simulink model "y003"  (R2019b)
settings: Solver=ode23tb  StartTime=0.0  StopTime=1  MaxStep=0.00001  RelTol=1e-3
values from neighbouring files (symbols this model uses):
  band = 0.01    [parameter.m]
  fN = 50    [parameter.m]
  J = 0.1284    [parameter.m]
  Llr = Lr - Lm    (= 0.006)    [parameter.m]
  Lls = Ls - Lm    (= 0.0102)    [parameter.m]
  np = 2    [parameter.m]
  PN = 3000    [parameter.m]
  Rr = 2.685    [parameter.m]
  Rs = 1.85    [parameter.m]
  TN = PN/(2*pi*nN/60)    (= 20.4627783975)    [parameter.m]
  UN = 380    [parameter.m]
undefined symbols (not defined in the file or in its folder): i
libraries: powerlib x9, simulink x3
Description:
  | 直接使用转子磁链数据，电流滞环跟踪
settings Model: Creator=Inspiron  LastModifiedBy=Inspiron
settings SolverCC: ZeroCrossAlgorithm=Adaptive
settings DebuggingCC: IgnoredZcDiagnostic=none

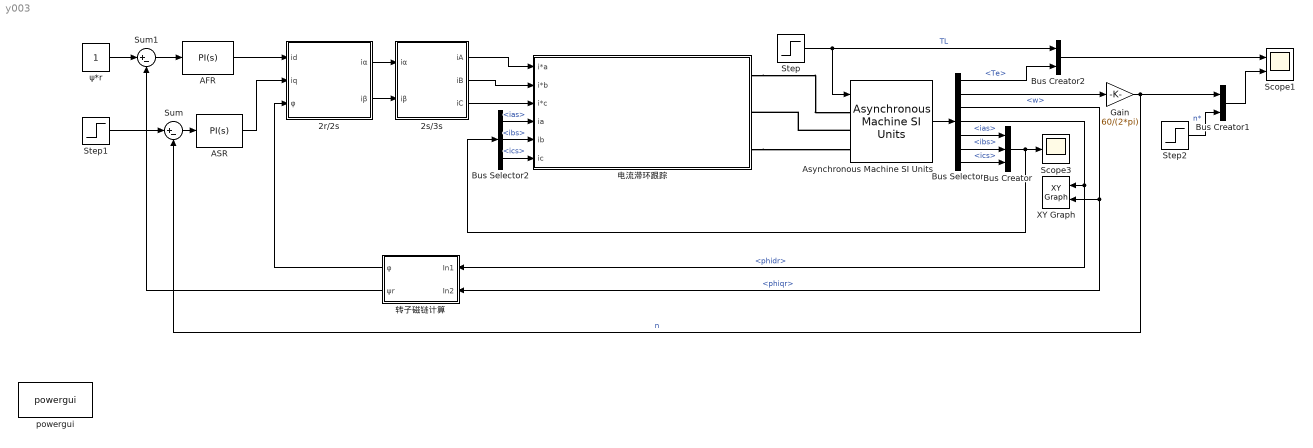
== system y003 ==
  2r/2s : Subsystem
  2s/3s : Subsystem
  AFR : simulink/Continuous/PID Controller  Controller=PI  Form=Parallel  TimeDomain=Continuous-time  SampleTime=-1  IntegratorMethod=Forward Euler  FilterMethod=Forward Euler  ControllerParametersSource=internal  P=80  I=20  D=0  UseFilter=on  N=100  TunerSelectOption=Transfer Function Based (PID Tuner App)  InitialConditionSource=internal  InitialConditionForIntegrator=0  InitialConditionForFilter=0  DifferentiatorICPrevScaledInput=0  ExternalReset=none  TrackingMode=off  Kt=1  LimitOutput=on  UpperSaturationLimit=40  LowerSaturationLimit=-40  LinearizeAsGain=on  AntiWindupMode=none  Kb=1  POutMin=[]  POutMax=[]  IOutMin=[]  IOutMax=[]  DOutMin=[]  DOutMax=[]  NOutMin=[]  NOutMax=[]  SumOutMin=[]  SumOutMax=[]  SaturationOutMin=[]  SaturationOutMax=[]  PParamMin=[]  PParamMax=[]  IParamMin=[]  IParamMax=[]  DParamMin=[]  DParamMax=[]  NParamMin=[]  NParamMax=[]  KbParamMin=[]  KbParamMax=[]  KtParamMin=[]  KtParamMax=[]  KbOutMin=[]  KbOutMax=[]  KtOutMin=[]  KtOutMax=[]  IntegratorOutMin=[]  IntegratorOutMax=[]  FilterOutMin=[]  FilterOutMax=[]  SumI1OutMin=[]  SumI1OutMax=[]  SumI2OutMin=[]  SumI2OutMax=[]  SumI3OutMin=[]  SumI3OutMax=[]  SumI4OutMin=[]  SumI4OutMax=[]  SumDOutMin=[]  SumDOutMax=[]  DifferentiatorOutMin=[]  DifferentiatorOutMax=[]  FilterDiffOutCoefMin=[]  FilterDiffOutCoefMax=[]  ReciprocalOutMin=[]  ReciprocalOutMax=[]  SumDenOutMin=[]  SumDenOutMax=[]  SumNumOutMin=[]  SumNumOutMax=[]  DivideOutMin=[]  DivideOutMax=[]  IntegratorContinuousStateAttributes=''  IntegratorStateMustResolveToSignalObject=off  IntegratorRTWStateStorageClass=Auto  FilterContinuousStateAttributes=''  FilterStateMustResolveToSignalObject=off  FilterRTWStateStorageClass=Auto  ParallelPVariant=InternalParameters  IdealPVariant=Disabled  IVariant=InternalParameters  DVariant=Disabled  IntegratorVariant=Continuous  SatVariant=Enabled  AWVariant=Passthrough  PCopyVariant=Disabled  TRVariant=Disabled  FdbkBlocksVariant=Forward  IdealPFdbkVariant=Disabled  SatFdbkVariant=Disabled  DerivativeFilterVariant=Disabled  NVariant=Disabled  NCopyVariant=Disabled_SignalSpec  FilterICVariant=Disabled  IntegratorICVariant=InternalICs  ExternalResetVariant=Disabled  TRSumVariant=Passthrough  SumFdbkVariant=Disabled  SumVariant=Sum_PI
  ASR : simulink/Continuous/PID Controller  Controller=PI  Form=Parallel  TimeDomain=Continuous-time  SampleTime=-1  IntegratorMethod=Forward Euler  FilterMethod=Forward Euler  ControllerParametersSource=internal  P=1  I=0.1  D=0  UseFilter=on  N=100  TunerSelectOption=Transfer Function Based (PID Tuner App)  InitialConditionSource=internal  InitialConditionForIntegrator=0  InitialConditionForFilter=0  DifferentiatorICPrevScaledInput=0  ExternalReset=none  TrackingMode=off  Kt=1  LimitOutput=on  UpperSaturationLimit=40  LowerSaturationLimit=-40  LinearizeAsGain=on  AntiWindupMode=none  Kb=1  POutMin=[]  POutMax=[]  IOutMin=[]  IOutMax=[]  DOutMin=[]  DOutMax=[]  NOutMin=[]  NOutMax=[]  SumOutMin=[]  SumOutMax=[]  SaturationOutMin=[]  SaturationOutMax=[]  PParamMin=[]  PParamMax=[]  IParamMin=[]  IParamMax=[]  DParamMin=[]  DParamMax=[]  NParamMin=[]  NParamMax=[]  KbParamMin=[]  KbParamMax=[]  KtParamMin=[]  KtParamMax=[]  KbOutMin=[]  KbOutMax=[]  KtOutMin=[]  KtOutMax=[]  IntegratorOutMin=[]  IntegratorOutMax=[]  FilterOutMin=[]  FilterOutMax=[]  SumI1OutMin=[]  SumI1OutMax=[]  SumI2OutMin=[]  SumI2OutMax=[]  SumI3OutMin=[]  SumI3OutMax=[]  SumI4OutMin=[]  SumI4OutMax=[]  SumDOutMin=[]  SumDOutMax=[]  DifferentiatorOutMin=[]  DifferentiatorOutMax=[]  FilterDiffOutCoefMin=[]  FilterDiffOutCoefMax=[]  ReciprocalOutMin=[]  ReciprocalOutMax=[]  SumDenOutMin=[]  SumDenOutMax=[]  SumNumOutMin=[]  SumNumOutMax=[]  DivideOutMin=[]  DivideOutMax=[]  IntegratorContinuousStateAttributes=''  IntegratorStateMustResolveToSignalObject=off  IntegratorRTWStateStorageClass=Auto  FilterContinuousStateAttributes=''  FilterStateMustResolveToSignalObject=off  FilterRTWStateStorageClass=Auto  ParallelPVariant=InternalParameters  IdealPVariant=Disabled  IVariant=InternalParameters  DVariant=Disabled  IntegratorVariant=Continuous  SatVariant=Enabled  AWVariant=Passthrough  PCopyVariant=Disabled  TRVariant=Disabled  FdbkBlocksVariant=Forward  IdealPFdbkVariant=Disabled  SatFdbkVariant=Disabled  DerivativeFilterVariant=Disabled  NVariant=Disabled  NCopyVariant=Disabled_SignalSpec  FilterICVariant=Disabled  IntegratorICVariant=InternalICs  ExternalResetVariant=Disabled  TRSumVariant=Passthrough  SumFdbkVariant=Disabled  SumVariant=Sum_PI
  Asynchronous Machine SI Units : powerlib/Machines/Asynchronous Machine SI Units  RotorType=Squirrel-cage  PresetModel=No  MechanicalLoad=Torque Tm  ShowDetailedParameters=on  ReferenceFrame=Stationary  Units=SI  MeasurementBus=on  NominalParameters=[PN UN fN]  Stator=[Rs Lls]  Rotor=[Rr Llr]  Cage1=[0.4155 0.002066]  Cage2=[0.4168 0.0003495]  Lm=Lm  Mechanical=[J 0 np]  PolePairs=2  InitialConditions=[1 0 0 0 0 0 0 0]  SimulateSaturation=off  Saturation=[14.03593122, 27.81365428, 53.79336849, 72.68890987, 97.98006896, 148.6815601, 215.7428561, 302.9841135, 428.7778367 ; 230, 322, 414, 460, 506, 552, 598, 644, 690]  LoadFlowParameters=1492000  TsPowergui=0  TsBlock=-1  IterativeModel=Trapezoidal non iterative  IterativeDiscreteModel=Trapezoidal non iterative  Pmec=1.492e+006
      settings: SourceProductName=Simscape Electrical
  Bus Creator : BusCreator  Inputs=3
  Bus Creator1 : BusCreator  Inputs=2
  Bus Creator2 : BusCreator  Inputs=2
  Bus Selector : BusSelector  OutputSignals=Te,w,phiqr,phidr,ias,ibs,ics
  Bus Selector2 : BusSelector  OutputSignals=ias,ibs,ics
  Gain : Gain  Gain=60/(2*pi)
  Scope1 : Scope  NumInputPorts=2
  Scope3 : Scope
  Step : Step  Time=0.4  After=TN  VectorParams1D=off  ZeroCross=off
  Step1 : Step  Time=0.6  Before=1000  After=0  SampleTime=0
  Step2 : Step  Time=0.6  Before=1000  After=0  SampleTime=0
  Sum : Sum  Inputs=|+-
  Sum1 : Sum  Inputs=|+-
  XY Graph : simulink/Sinks/XY Graph  xmin=-2  xmax=2  ymin=-2  ymax=2  st=-1
  powergui : powerlib/powergui  Priority=1  SimulationMode=Discrete  SampleTime=1e-5  frequency=60  Iterations=50  frequencyindice=50  Pbase=100e6  ErrMax=1e-4  UnitsV=kV  UnitsW=MW  buscounter=0  FunctionMessages=off  echomessages=off  EnableUseOfTLC=off  CurrentSourceSwitches=off  DisableSnubberDevices=off  DisableRonSwitches=off  DisableVfSwitches=off  DisplayEquations=off  AutomaticDiscreteSolvers=off  SolverType=Tustin/Backward Euler (TBE)  Interpol=off  ExternalGateDelay=off  methode=off  Ts=100  x0status=blocks  SPID=on  SwTol=0  HookPort=off  NonlinearTolerance=1e-4  nMaxIteration=100  ContinueOnMaxIteration=off  RestoreLinks=warning  ResistiveCurrentMeasurement=off  Frange=[0:2:500]  Ylog=off  Xlog=on  ShowGrid=off  save=off  variable=ZData  structure=0  ZoomFFT=off  StartTime=0.0  cycles=1  DisplayStyle=1  fundamental=60  FreqAxis=off  MaxFrequency=1000  frequencyindicesteady=1  RmsSteady=1  display=off
      settings: SourceProductName=Simscape Electrical
  ψ*r : Constant
  电流滞环跟踪 : Subsystem
  转子磁链计算 : Subsystem
  wires:
  Asynchronous Machine SI Units/1 -> Bus Selector/1
  Bus Creator/1 -> Scope3/1, Bus Selector2/1
  Gain/1 -> Bus Creator1/1, Sum/2  "n"
  Bus Selector/2 -> Gain/1  "<w>"
  Bus Selector/5 -> Bus Creator/1  "<ias>"
  Bus Selector/6 -> Bus Creator/2  "<ibs>"
  Bus Selector/7 -> Bus Creator/3  "<ics>"
  Bus Selector/3 -> 转子磁链计算/2(In2), XY Graph/2  "<phiqr>"
  Bus Selector/4 -> 转子磁链计算/1(In1), XY Graph/1  "<phidr>"
  2r/2s/1(iα) -> 2s/3s/1(iα)
  2r/2s/2(iβ) -> 2s/3s/2(iβ)
  Bus Selector2/1 -> 电流滞环跟踪/4(ia)  "<ias>"
  Bus Selector2/2 -> 电流滞环跟踪/5(ib)  "<ibs>"
  Bus Selector2/3 -> 电流滞环跟踪/6(ic)  "<ics>"
  2s/3s/1(iA) -> 电流滞环跟踪/1(i*a)
  2s/3s/2(iB) -> 电流滞环跟踪/2(i*b)
  2s/3s/3(iC) -> 电流滞环跟踪/3(i*c)
  Step1/1 -> Sum/1
  Sum/1 -> ASR/1
  ASR/1 -> 2r/2s/2(iq)
  ψ*r/1 -> Sum1/1
  Sum1/1 -> AFR/1
  AFR/1 -> 2r/2s/1(id)
  转子磁链计算/2(ψr) -> Sum1/2
  转子磁链计算/1(φ) -> 2r/2s/3(φ)
  Step/1 -> Asynchronous Machine SI Units/1, Bus Creator2/1  "TL"
  Step2/1 -> Bus Creator1/2  "n*"
  Bus Selector/1 -> Bus Creator2/2  "<Te>"
  Bus Creator2/1 -> Scope1/1
  Bus Creator1/1 -> Scope1/2
  connections:
  电流滞环跟踪/RConn3 -- Asynchronous Machine SI Units/LConn3
  Asynchronous Machine SI Units/LConn2 -- 电流滞环跟踪/RConn2
  电流滞环跟踪/RConn1 -- Asynchronous Machine SI Units/LConn1

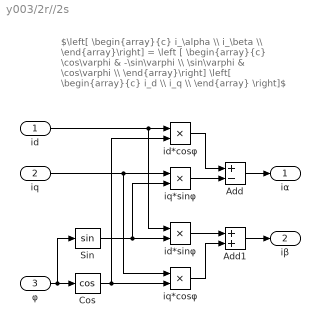
== system y003/2r//2s ==
  note: $\left[ \begin{array}{c} i_\alpha \\ i_\beta \\ \end{array}\right] = \left [ \begin{array}{c} \cos\varphi & -\sin\varphi \\ \sin\varphi & \cos\varphi \\ \end{array}\right] \left[ \begin{array}{c} i_d \\ i_q \\ \end{array} \right]$
  id : Inport
  iq : Inport  Port=2
  φ : Inport  Port=3
  Add : Sum  Inputs=+-
  Add1 : Sum
  Cos : Trigonometry  Operator=cos
  Sin : Trigonometry
  id*cosφ : Product
  id*sinφ : Product
  iq*cosφ : Product
  iq*sinφ : Product
  iα : Outport
  iβ : Outport  Port=2
  wires:
  Cos/1 -> iq*cosφ/2, id*cosφ/2
  iq*cosφ/1 -> Add1/2
  Sin/1 -> id*sinφ/2, iq*sinφ/2
  id/1 -> id*cosφ/1, id*sinφ/1
  id*sinφ/1 -> Add1/1
  iq*sinφ/1 -> Add/2
  iq/1 -> iq*sinφ/1, iq*cosφ/1
  φ/1 -> Sin/1, Cos/1
  Add/1 -> iα/1
  id*cosφ/1 -> Add/1
  Add1/1 -> iβ/1

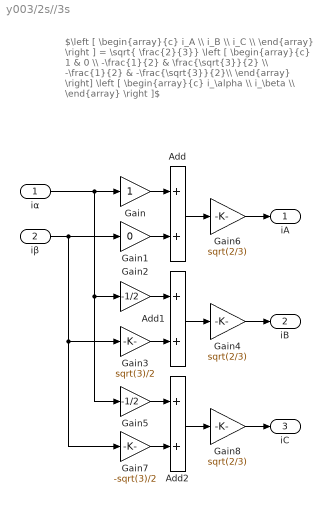
== system y003/2s//3s ==
  note: $\left [ \begin{array}{c} i_A \\ i_B \\ i_C \\ \end{array} \right ] = \sqrt{ \frac{2}{3}} \left [ \begin{array}{c} 1 & 0 \\ -\frac{1}{2} & \frac{\sqrt{3}}{2} \\ -\frac{1}{2} & -\frac{\sqrt{3}}{2}\\ \end{array} \right] \left [ \begin{array}{c} i_\alpha \\ i_\beta \\ \end{array} \right ]$
  iα : Inport
  iβ : Inport  Port=2
  Add : Sum  Inputs=2
  Add1 : Sum  Inputs=2
  Add2 : Sum  Inputs=2
  Gain : Gain
  Gain1 : Gain  Gain=0
  Gain2 : Gain  Gain=-1/2
  Gain3 : Gain  Gain=sqrt(3)/2
  Gain4 : Gain  Gain=sqrt(2/3)
  Gain5 : Gain  Gain=-1/2
  Gain6 : Gain  Gain=sqrt(2/3)
  Gain7 : Gain  Gain=-sqrt(3)/2
  Gain8 : Gain  Gain=sqrt(2/3)
  iA : Outport
  iB : Outport  Port=2
  iC : Outport  Port=3
  wires:
  Gain/1 -> Add/1
  iβ/1 -> Gain7/1, Gain3/1, Gain1/1
  Add/1 -> Gain6/1
  Gain1/1 -> Add/2
  iα/1 -> Gain5/1, Gain2/1, Gain/1
  Gain4/1 -> iB/1
  Gain6/1 -> iA/1
  Gain2/1 -> Add1/1
  Gain3/1 -> Add1/2
  Add1/1 -> Gain4/1
  Gain5/1 -> Add2/1
  Gain7/1 -> Add2/2
  Gain8/1 -> iC/1
  Add2/1 -> Gain8/1

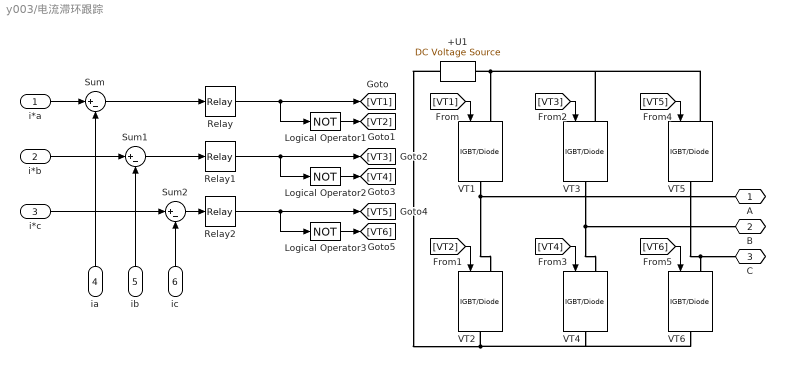
== system y003/电流滞环跟踪 ==
  i*a : Inport
  i*b : Inport  Port=2
  i*c : Inport  Port=3
  ia : Inport  Port=4
  ib : Inport  Port=5
  ic : Inport  Port=6
  +U1 : powerlib/Electrical Sources/DC Voltage Source  Amplitude=510  Measurements=None
      settings: SourceProductName=Simscape Electrical
  Logical Operator1 : Logic  Operator=NOT  AllPortsSameDT=off  OutDataTypeStr=boolean
  Logical Operator2 : Logic  Operator=NOT  AllPortsSameDT=off  OutDataTypeStr=boolean
  Logical Operator3 : Logic  Operator=NOT  AllPortsSameDT=off  OutDataTypeStr=boolean
  Relay : Relay  OnSwitchValue=band  OffSwitchValue=-band
  Relay1 : Relay  OnSwitchValue=band  OffSwitchValue=-band
  Relay2 : Relay  OnSwitchValue=band  OffSwitchValue=-band
  Sum : Sum  Inputs=|+-
  Sum1 : Sum  Inputs=|+-
  Sum2 : Sum  Inputs=|+-
  VT{1..6} (6 alike) : powerlib/Power Electronics/IGBT//Diode  Ron=1e-3  Rs=1e5  Cs=inf  Measurements=off
      settings: SourceProductName=Simscape Electrical
  A : PMIOPort  Side=Right
  B : PMIOPort  Port=2  Side=Right
  C : PMIOPort  Port=3  Side=Right
  wires:
  [VT3] -> VT3/1
  Relay/1 -> Logical Operator1/1, [VT1]
  [VT4] -> VT4/1
  Sum2/1 -> Relay2/1
  Relay1/1 -> Logical Operator2/1, [VT3]
  ic/1 -> Sum2/2
  Sum/1 -> Relay/1
  Sum1/1 -> Relay1/1
  [VT5] -> VT5/1
  Logical Operator3/1 -> [VT6]
  Relay2/1 -> Logical Operator3/1, [VT5]
  i*c/1 -> Sum2/1
  ia/1 -> Sum/2
  Logical Operator2/1 -> [VT4]
  [VT6] -> VT6/1
  [VT2] -> VT2/1
  Logical Operator1/1 -> [VT2]
  [VT1] -> VT1/1
  ib/1 -> Sum1/2
  i*a/1 -> Sum/1
  i*b/1 -> Sum1/1
  connections:
  +U1/RConn1 -- VT3/LConn1 -- VT5/LConn1 -- VT1/LConn1
  VT6/RConn1 -- VT4/RConn1 -- +U1/LConn1 -- VT2/RConn1
  VT5/RConn1 -- C/RConn1 -- VT6/LConn1
  VT3/RConn1 -- VT4/LConn1 -- B/RConn1
  VT1/RConn1 -- VT2/LConn1 -- A/RConn1

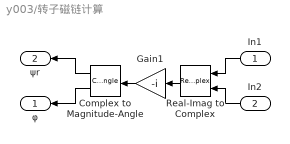
== system y003/转子磁链计算 ==
  In1 : Inport
  In2 : Inport  Port=2
  Complex to Magnitude-Angle : ComplexToMagnitudeAngle
  Gain1 : Gain  Gain=-i
  Real-Imag to Complex : RealImagToComplex
  φ : Outport
  ψr : Outport  Port=2
  wires:
  Gain1/1 -> Complex to Magnitude-Angle/1
  Real-Imag to Complex/1 -> Gain1/1
  In2/1 -> Real-Imag to Complex/2
  In1/1 -> Real-Imag to Complex/1
  Complex to Magnitude-Angle/2 -> φ/1
  Complex to Magnitude-Angle/1 -> ψr/1
